simulink model "model"  (R2020b)
settings: Solver=VariableStepAuto  StartTime=0.0  StopTime=10.0  RelTol=1e-3
undefined symbols (not defined in the file or in its folder): be, bv, Ie, lv, R, Uk
settings Model: DataDictionary=model_data_dictionary.sldd  Creator=Arvind Hishikar  LastModifiedBy=Arvind Hishikar

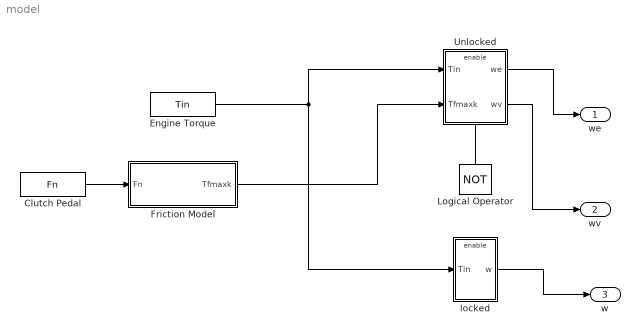
== system model ==
  Clutch Pedal : FromWorkspace  VariableName=Fn  ZeroCross=off
  Engine Torque : FromWorkspace  VariableName=Tin  ZeroCross=off
  Friction Model : Subsystem
  Logical Operator : Logic  Operator=NOT  IconShape=distinctive  AllPortsSameDT=off  OutDataTypeStr=boolean
  Unlocked : Subsystem
  locked : Subsystem
  we : Outport
  wv : Outport  Port=2
  w : Outport  Port=3
  wires:
  Clutch Pedal/1 -> Friction Model/1(Fn)
  Friction Model/1(Tfmaxk) -> Unlocked/2(Tfmaxk)
  Unlocked/1(we) -> we/1
  Unlocked/2(wv) -> wv/1
  Engine Torque/1 -> locked/1(Tin), Unlocked/1(Tin)
  locked/1(w) -> w/1
  Logical Operator/1 -> Unlocked/Enable
  ? -> Logical Operator/1, locked/Enable

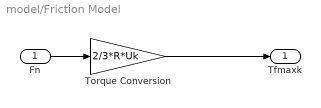
== system model/Friction Model ==
  Fn : Inport
  Torque Conversion : Gain  Gain=2/3*R*Uk
  Tfmaxk : Outport
  wires:
  Fn/1 -> Torque Conversion/1
  Torque Conversion/1 -> Tfmaxk/1

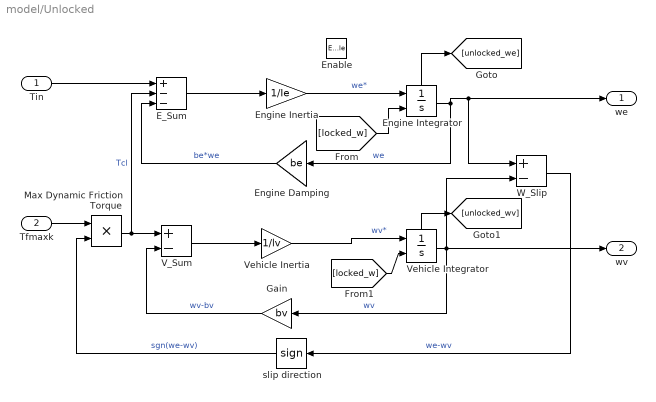
== system model/Unlocked ==
  Tin : Inport
  Tfmaxk : Inport  Port=2
  Enable : EnablePort  StatesWhenEnabling=reset
  E_Sum : Sum  Inputs=+--
  Engine Damping : Gain  Gain=be
  Engine Inertia : Gain  Gain=1/Ie
  Engine Integrator : Integrator  InitialConditionSource=external  ShowStatePort=on
  Gain : Gain  Gain=bv
  Max Dynamic Friction Torque : Product
  V_Sum : Sum  Inputs=+-
  Vehicle Inertia : Gain  Gain=1/lv
  Vehicle Integrator : Integrator  InitialConditionSource=external  ShowStatePort=on
  W_Slip : Sum  Inputs=+-
  slip direction : Signum
  we : Outport
  wv : Outport  Port=2
  wires:
  E_Sum/1 -> Engine Inertia/1
  Vehicle Integrator/1 -> W_Slip/2, wv/1, Gain/1  "wv"
  Vehicle Inertia/1 -> Vehicle Integrator/1  "wv*"
  Engine Damping/1 -> E_Sum/3  "be*we"
  W_Slip/1 -> slip direction/1  "we-wv"
  V_Sum/1 -> Vehicle Inertia/1
  Gain/1 -> V_Sum/2  "wv-bv"
  Engine Integrator/1 -> we/1, W_Slip/1, Engine Damping/1  "we"
  Tfmaxk/1 -> Max Dynamic Friction Torque/1
  Max Dynamic Friction Torque/1 -> V_Sum/1, E_Sum/2  "Tcl"
  slip direction/1 -> Max Dynamic Friction Torque/2  "sgn(we-wv)"
  Engine Inertia/1 -> Engine Integrator/1  "we*"
  Tin/1 -> E_Sum/1
  [locked_w] -> Engine Integrator/2
  Engine Integrator/State -> [unlocked_we]
  [locked_w] -> Vehicle Integrator/2
  Vehicle Integrator/State -> [unlocked_wv]

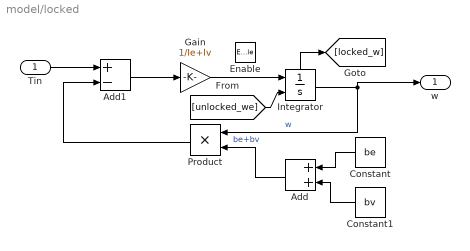
== system model/locked ==
  Tin : Inport
  Enable : EnablePort
  Add : Sum
  Add1 : Sum  Inputs=+-
  Constant : Constant  Value=be
  Constant1 : Constant  Value=bv
  Gain : Gain  Gain=1/Ie+lv
  Integrator : Integrator  InitialConditionSource=external  ShowStatePort=on
  Product : Product
  w : Outport
  wires:
  Product/1 -> Add1/2
  Tin/1 -> Add1/1
  Add1/1 -> Gain/1
  Integrator/1 -> w/1, Product/1  "w"
  Add/1 -> Product/2  "be+bv"
  Gain/1 -> Integrator/1
  Constant1/1 -> Add/2
  Constant/1 -> Add/1
  [unlocked_we] -> Integrator/2
  Integrator/State -> [locked_w]
